simulink model "panxuan"  (R2016a)
settings: Solver=VariableStepAuto  StartTime=0.0  StopTime=2000  RelTol=1e-3
undefined symbols (not defined in the file): A, B, C, D
libraries: simulink x2
settings Model: Creator=Gray  LastModifiedBy=Gray

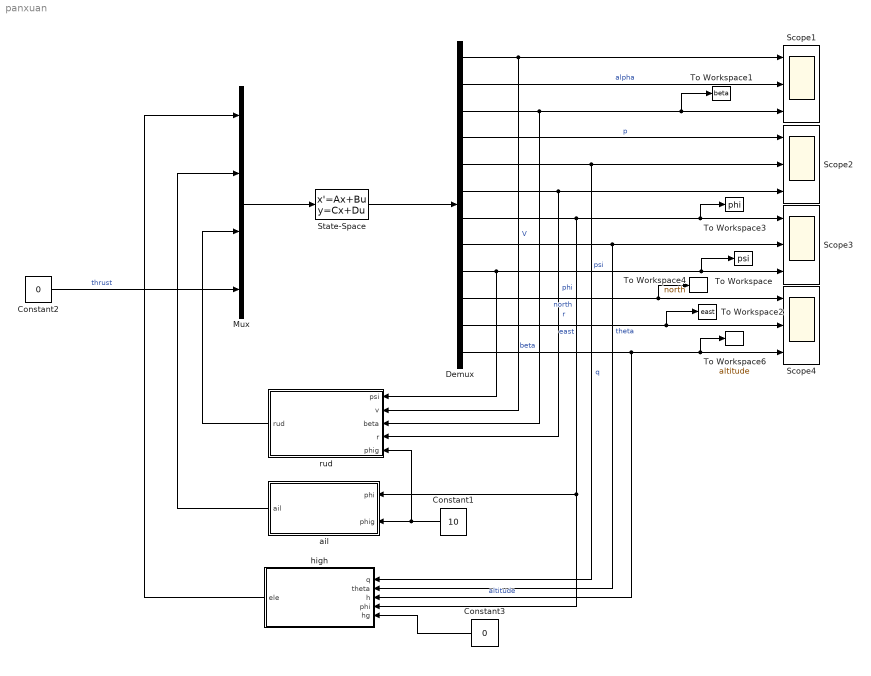
== system panxuan ==
  Constant1 : Constant  Value=10
  Constant2 : Constant  Value=0
  Constant3 : Constant  Value=0
  Demux : Demux  Outputs=12
  Mux : Mux
  Scope{1..4} (4 alike) : Scope  NumInputPorts=3
  State-Space : StateSpace  A=A  B=B  C=C  D=D  X0=[20 0 0 0 0 0 0 0 0 0 0 0]
  To Workspace : ToWorkspace  VariableName=psi  SaveFormat=Timeseries  SampleTime=-1
  To Workspace1 : ToWorkspace  VariableName=beta  SaveFormat=Timeseries  SampleTime=-1
  To Workspace2 : ToWorkspace  VariableName=east  SampleTime=-1
  To Workspace3 : ToWorkspace  VariableName=phi  SaveFormat=Timeseries  SampleTime=-1
  To Workspace4 : ToWorkspace  VariableName=north  SampleTime=-1
  To Workspace6 : ToWorkspace  VariableName=altitude  SaveFormat=Timeseries  SampleTime=-1
  ail : Subsystem
  "high " : Subsystem
  rud : Subsystem
  wires:
  State-Space/1 -> Demux/1
  Mux/1 -> State-Space/1
  Demux/1 -> rud/2(v), Scope1/1  "V"
  Demux/2 -> Scope1/2  "alpha"
  Demux/3 -> rud/3(beta), To Workspace1/1, Scope1/3  "beta"
  Demux/4 -> Scope2/1  "p"
  Demux/5 -> "high "/1(q), Scope2/2  "q"
  Demux/6 -> rud/4(r), Scope2/3  "r"
  Demux/7 -> "high "/4(phi), ail/1(phi), To Workspace3/1, Scope3/1  "phi"
  Demux/8 -> "high "/2(theta), Scope3/2  "theta"
  Demux/9 -> rud/1(psi), To Workspace/1, Scope3/3  "psi"
  Demux/10 -> To Workspace4/1, Scope4/1  "north"
  Demux/11 -> To Workspace2/1, Scope4/2  "east"
  Demux/12 -> "high "/3(h), To Workspace6/1, Scope4/3  "altitude"
  ail/1(ail) -> Mux/2
  Constant2/1 -> Mux/4  "thrust"
  Constant1/1 -> rud/5(phig), ail/2(phig)
  rud/1(rud) -> Mux/3
  Constant3/1 -> "high "/5(hg)
  "high "/1(ele) -> Mux/1

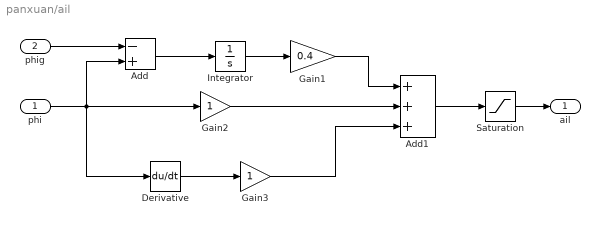
== system panxuan/ail ==
  phi : Inport
  phig : Inport  Port=2
  Add : Sum  Inputs=-+
  Add1 : Sum  Inputs=+++
  Derivative : Derivative
  Gain1 : Gain  Gain=0.4
  Gain2 : Gain
  Gain3 : Gain
  Integrator : Integrator
  Saturation : Saturate  UpperLimit=12  LowerLimit=-12
  ail : Outport
  wires:
  phi/1 -> Derivative/1, Add/2, Gain2/1
  Add1/1 -> Saturation/1
  Add/1 -> Integrator/1
  Integrator/1 -> Gain1/1
  Saturation/1 -> ail/1
  phig/1 -> Add/1
  Derivative/1 -> Gain3/1
  Gain2/1 -> Add1/2
  Gain3/1 -> Add1/3
  Gain1/1 -> Add1/1

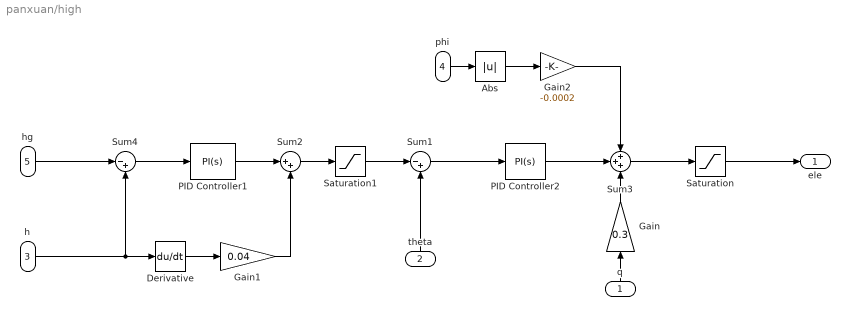
== system panxuan/high  ==
  q : Inport
  theta : Inport  Port=2
  h : Inport  Port=3
  phi : Inport  Port=4
  hg : Inport  Port=5
  Abs : Abs
  Derivative : Derivative
  Gain : Gain  Gain=0.3
  Gain1 : Gain  Gain=0.04
  Gain2 : Gain  Gain=-0.0002
  PID Controller1 : simulink/Continuous/PID Controller  Controller=PI  TimeDomain=Continuous-time  SampleTime=-1  IntegratorMethod=Forward Euler  FilterMethod=Forward Euler  Form=Parallel  UseFilter=on  ControllerParametersSource=internal  P=0.03  I=0.0002  D=0  N=100  InitialConditionSource=internal  InitialConditionForIntegrator=0  InitialConditionForFilter=0  ExternalReset=none  LimitOutput=off  UpperSaturationLimit=inf  LowerSaturationLimit=-inf  LinearizeAsGain=on  AntiWindupMode=none  Kb=1  TrackingMode=off  Kt=1  PParamMin=[]  PParamMax=[]  IParamMin=[]  IParamMax=[]  DParamMin=[]  DParamMax=[]  NParamMin=[]  NParamMax=[]  KbParamMin=[]  KbParamMax=[]  KtParamMin=[]  KtParamMax=[]  POutMin=[]  POutMax=[]  IOutMin=[]  IOutMax=[]  DOutMin=[]  DOutMax=[]  NOutMin=[]  NOutMax=[]  KbOutMin=[]  KbOutMax=[]  KtOutMin=[]  KtOutMax=[]  IntegratorOutMin=[]  IntegratorOutMax=[]  FilterOutMin=[]  FilterOutMax=[]  SumOutMin=[]  SumOutMax=[]  SumI1OutMin=[]  SumI1OutMax=[]  SumI2OutMin=[]  SumI2OutMax=[]  SumI3OutMin=[]  SumI3OutMax=[]  SumDOutMin=[]  SumDOutMax=[]  SaturationOutMin=[]  SaturationOutMax=[]  IntegratorContinuousStateAttributes=''  IntegratorStateMustResolveToSignalObject=off  IntegratorRTWStateStorageClass=Auto  FilterContinuousStateAttributes=''  FilterStateMustResolveToSignalObject=off  FilterRTWStateStorageClass=Auto  DifferentiatorICPrevScaledInput=0  DifferentiatorOutMin=[]  DifferentiatorOutMax=[]
  PID Controller2 : simulink/Continuous/PID Controller  Controller=PI  TimeDomain=Continuous-time  SampleTime=-1  IntegratorMethod=Forward Euler  FilterMethod=Forward Euler  Form=Parallel  UseFilter=on  ControllerParametersSource=internal  P=0.5  I=0  D=0  N=100  InitialConditionSource=internal  InitialConditionForIntegrator=0  InitialConditionForFilter=0  ExternalReset=none  LimitOutput=off  UpperSaturationLimit=inf  LowerSaturationLimit=-inf  LinearizeAsGain=on  AntiWindupMode=none  Kb=1  TrackingMode=off  Kt=1  PParamMin=[]  PParamMax=[]  IParamMin=[]  IParamMax=[]  DParamMin=[]  DParamMax=[]  NParamMin=[]  NParamMax=[]  KbParamMin=[]  KbParamMax=[]  KtParamMin=[]  KtParamMax=[]  POutMin=[]  POutMax=[]  IOutMin=[]  IOutMax=[]  DOutMin=[]  DOutMax=[]  NOutMin=[]  NOutMax=[]  KbOutMin=[]  KbOutMax=[]  KtOutMin=[]  KtOutMax=[]  IntegratorOutMin=[]  IntegratorOutMax=[]  FilterOutMin=[]  FilterOutMax=[]  SumOutMin=[]  SumOutMax=[]  SumI1OutMin=[]  SumI1OutMax=[]  SumI2OutMin=[]  SumI2OutMax=[]  SumI3OutMin=[]  SumI3OutMax=[]  SumDOutMin=[]  SumDOutMax=[]  SaturationOutMin=[]  SaturationOutMax=[]  IntegratorContinuousStateAttributes=''  IntegratorStateMustResolveToSignalObject=off  IntegratorRTWStateStorageClass=Auto  FilterContinuousStateAttributes=''  FilterStateMustResolveToSignalObject=off  FilterRTWStateStorageClass=Auto  DifferentiatorICPrevScaledInput=0  DifferentiatorOutMin=[]  DifferentiatorOutMax=[]
  Saturation : Saturate  UpperLimit=9  LowerLimit=-9
  Saturation1 : Saturate  UpperLimit=15  LowerLimit=-15
  Sum1 : Sum  Inputs=|-+
  Sum2 : Sum  Inputs=|++
  Sum3 : Sum  Inputs=+++
  Sum4 : Sum  Inputs=|-+
  ele : Outport
  wires:
  hg/1 -> Sum4/1
  Sum4/1 -> PID Controller1/1
  PID Controller1/1 -> Sum2/1
  Sum1/1 -> PID Controller2/1
  Sum3/1 -> Saturation/1
  h/1 -> Derivative/1, Sum4/2
  theta/1 -> Sum1/2
  q/1 -> Gain/1
  Saturation/1 -> ele/1
  Saturation1/1 -> Sum1/1
  Sum2/1 -> Saturation1/1
  Derivative/1 -> Gain1/1
  Gain1/1 -> Sum2/2
  PID Controller2/1 -> Sum3/2
  Gain/1 -> Sum3/3
  phi/1 -> Abs/1
  Abs/1 -> Gain2/1
  Gain2/1 -> Sum3/1

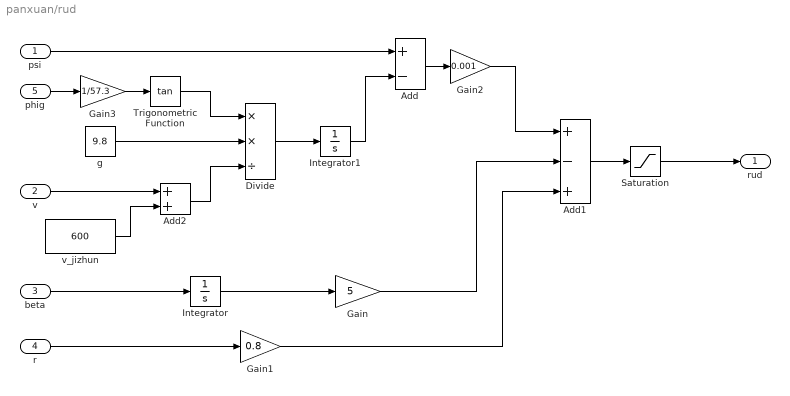
== system panxuan/rud ==
  psi : Inport
  v : Inport  Port=2
  beta : Inport  Port=3
  r : Inport  Port=4
  phig : Inport  Port=5
  Add : Sum  Inputs=+-
  Add1 : Sum  Inputs=+-+
  Add2 : Sum
  Divide : Product  Inputs=**/
  Gain : Gain  Gain=5
  Gain1 : Gain  Gain=0.8
  Gain2 : Gain  Gain=0.001
  Gain3 : Gain  Gain=1/57.3
  Integrator : Integrator
  Integrator1 : Integrator
  Saturation : Saturate  UpperLimit=8  LowerLimit=-8
  Trigonometric Function : Trigonometry  Operator=tan
  g : Constant  Value=9.8
  v_jizhun : Constant  Value=600
  rud : Outport
  wires:
  Saturation/1 -> rud/1
  Add1/1 -> Saturation/1
  Trigonometric Function/1 -> Divide/1
  g/1 -> Divide/2
  psi/1 -> Add/1
  Add/1 -> Gain2/1
  r/1 -> Gain1/1
  Divide/1 -> Integrator1/1
  Integrator1/1 -> Add/2
  Add2/1 -> Divide/3
  v/1 -> Add2/1
  v_jizhun/1 -> Add2/2
  Gain1/1 -> Add1/3
  Integrator/1 -> Gain/1
  beta/1 -> Integrator/1
  Gain2/1 -> Add1/1
  Gain/1 -> Add1/2
  phig/1 -> Gain3/1
  Gain3/1 -> Trigonometric Function/1
